simulink model "EMPlanner_cs_old"  (R2020a)
settings: Solver=ode5  StartTime=0.0  StopTime=120  FixedStep=1/1000  RelTol=1e-3
PreLoadFcn:
  | mbxruntime.callbacks.PreLoadFcn(bdroot);
PostLoadFcn:
  | mbxruntime.callbacks.PostLoadFcn(bdroot);
InitFcn:
  | mbxruntime.callbacks.InitFcn(bdroot);
StartFcn:
  | mbxruntime.callbacks.StartFcn(bdroot);
StopFcn:
  | mbxruntime.callbacks.StopFcn(bdroot);
model workspace (MAT data in the model file):
  mbox_table : object (value not decoded)
  model_closed = 0
  sim_status = 0
values from neighbouring files (symbols this model uses):
  c_factor = 43.75    [emplanner_init.m]
  cf = -175016    [emplanner_init.m]
  cr = -130634    [emplanner_init.m]
  KD_PID_distance = 0.0    (= 0)    [emplanner_init.m]
  KD_PID_speed = 0    [emplanner_init.m]
  KI_PID_distance = 0.0    (= 0)    [emplanner_init.m]
  KI_PID_speed = 0    [emplanner_init.m]
  KP_PID_distance = 0.5    [emplanner_init.m]
  KP_PID_speed = 1.8    [emplanner_init.m]
  la = 1.265    [emplanner_init.m]
  lb = 2.947-1.265    (= 1.682)    [emplanner_init.m]
  LQR_K1 = k(:,1)'    [emplanner_init.m]
  LQR_K2 = k(:,2)'    [emplanner_init.m]
  LQR_K3 = k(:,3)'    [emplanner_init.m]
  LQR_K4 = k(:,4)'    [emplanner_init.m]
  m = 2020    [emplanner_init.m]
  rack_displacement = [-39.14 , -37.2 , -35.29 , -33.43 , -31.6 , -29.81 , -28.06 , -26.34 , -24.66 ,      -23.01 , -21.38 , -19.79 , -18.23 , -16.69 , -15.18 , -13.7 , -12.23 , -10.8 , -9.38 , -7.98 ,     -6.61 , -5.25 , -3.91 , -2.59 , -1.29 , 0 , 1.27 , 2.54 , 3.78 , 5.02 , 6.24 , 7.46 , 8.66 ,      9.86 , 11.05 , 12.24 , 13.41 , 14.59 , 15.76 , 16.92 , 18.09 , 19.25 , 20.42 , 21.59 , 22.76 ,      23.93 , 25.11 , 26 ...(+26 chars)    [emplanner_init.m]
  right_wheel_ground = [-70 ,-67.2 , -64.4 , -61.6 , -58.8 , -56 , -53.2 , -50.4 , -47.6 , -44.8 , -42 ,      -39.2 , -36.4 , -33.6 , -30.8 , -28 , -25.2 , -22.4 , -19.6 , -16.8 , -14 , -11.2 , -8.4 , -5.6 ,      -2.8 , 0 , 2.8 , 5.6 , 8.4 , 11.2 , 14 , 16.8 , 19.6 , 22.4 , 25.2 , 28 , 30.8 , 33.6 , 36.4 ,      39.2 , 42 , 44.8 , 47.6 , 50.4 , 53.2 , 56 , 58.8 , 61.6 , 64.4 , 67.2 , 70 ]    [emplanner_init.m]
  vx_break_point = zeros(1,5000)    [emplanner_init.m]
undefined symbols (not defined in the file or in its folder): aubr, DiscIntNeverNeededParam, global_path_x, global_path_y, tablebr, vubr, warningInitialVelocity, x0
libraries: PreScanSimulinkLibrary x21, simulink x19, simulink_extras x6, Solver_SF x1
(part 4 of 9)

== system EMPlanner_cs_old/Audi_A8_Sedan_1/AIR_1_Demux/Activate_Switch ==
  BeamID : Inport
  Heading : Inport  Port=2
  Constant : Constant  Value=0
  Product1 : Product  RndMeth=Zero
  Relational Operator : RelationalOperator  Operator=~=  OutDataTypeStr=boolean  RndMeth=Nearest
  On/Off : Outport
  wires:
  Constant/1 -> Relational Operator/1
  Relational Operator/1 -> Product1/1
  BeamID/1 -> Relational Operator/2
  Product1/1 -> On/Off/1
  Heading/1 -> Product1/2

== system EMPlanner_cs_old/Audi_A8_Sedan_1/AIR_1_Demux/Signal2ArrayOfSignals1 ==
  note: Set mask parameter VECTORLENGTH
      |  to MAXMESSAGES
  note: Initial state of Previous vector block
      | set to zeros(VECTORLENGTH,1)
  LoopIndex : Inport
  Element : Inport  Port=2
  Assignment : Assignment  IndexOptions=Index vector (port)  Indices=1  OutputSizes=1
  Previous vector : Memory  InitialCondition=zeros(VECTORLENGTH,1)  InheritSampleTime=on
  ArrayofElements : Outport
  wires:
  Element/1 -> Assignment/2
  LoopIndex/1 -> Assignment/3
  Previous vector/1 -> Assignment/1
  Assignment/1 -> ArrayofElements/1, Previous vector/1

== system EMPlanner_cs_old/Audi_A8_Sedan_1/AIR_1_Demux/Signal2ArrayOfSignals2 ==
  note: Set mask parameter VECTORLENGTH
      |  to MAXMESSAGES
  note: Initial state of Previous vector block
      | set to zeros(VECTORLENGTH,1)
  LoopIndex : Inport
  Element : Inport  Port=2
  Assignment : Assignment  IndexOptions=Index vector (port)  Indices=1  OutputSizes=1
  Previous vector : Memory  InitialCondition=zeros(VECTORLENGTH,1)  InheritSampleTime=on
  ArrayofElements : Outport
  wires:
  Element/1 -> Assignment/2
  LoopIndex/1 -> Assignment/3
  Previous vector/1 -> Assignment/1
  Assignment/1 -> ArrayofElements/1, Previous vector/1

== system EMPlanner_cs_old/Audi_A8_Sedan_1/AIR_1_Demux/Signal2ArrayOfSignals3 ==
  note: Set mask parameter VECTORLENGTH
      |  to MAXMESSAGES
  note: Initial state of Previous vector block
      | set to zeros(VECTORLENGTH,1)
  LoopIndex : Inport
  Element : Inport  Port=2
  Assignment : Assignment  IndexOptions=Index vector (port)  Indices=1  OutputSizes=1
  Previous vector : Memory  InitialCondition=zeros(VECTORLENGTH,1)  InheritSampleTime=on
  ArrayofElements : Outport
  wires:
  Element/1 -> Assignment/2
  LoopIndex/1 -> Assignment/3
  Previous vector/1 -> Assignment/1
  Assignment/1 -> ArrayofElements/1, Previous vector/1

== system EMPlanner_cs_old/Audi_A8_Sedan_1/AIR_1_Demux/Signal2ArrayOfSignals4 ==
  note: Set mask parameter VECTORLENGTH
      |  to MAXMESSAGES
  note: Initial state of Previous vector block
      | set to zeros(VECTORLENGTH,1)
  LoopIndex : Inport
  Element : Inport  Port=2
  Assignment : Assignment  IndexOptions=Index vector (port)  Indices=1  OutputSizes=1
  Previous vector : Memory  InitialCondition=zeros(VECTORLENGTH,1)  InheritSampleTime=on
  ArrayofElements : Outport
  wires:
  Element/1 -> Assignment/2
  LoopIndex/1 -> Assignment/3
  Previous vector/1 -> Assignment/1
  Assignment/1 -> ArrayofElements/1, Previous vector/1

== system EMPlanner_cs_old/Audi_A8_Sedan_1/AIR_1_Demux/Signal2ArrayOfSignals5 ==
  note: Set mask parameter VECTORLENGTH
      |  to MAXMESSAGES
  note: Initial state of Previous vector block
      | set to zeros(VECTORLENGTH,1)
  LoopIndex : Inport
  Element : Inport  Port=2
  Assignment : Assignment  IndexOptions=Index vector (port)  Indices=1  OutputSizes=1
  Previous vector : Memory  InitialCondition=zeros(VECTORLENGTH,1)  InheritSampleTime=on
  ArrayofElements : Outport
  wires:
  Element/1 -> Assignment/2
  LoopIndex/1 -> Assignment/3
  Previous vector/1 -> Assignment/1
  Assignment/1 -> ArrayofElements/1, Previous vector/1

== system EMPlanner_cs_old/Audi_A8_Sedan_1/AIR_1_Demux/Signal2ArrayOfSignals6 ==
  note: Set mask parameter VECTORLENGTH
      |  to MAXMESSAGES
  note: Initial state of Previous vector block
      | set to zeros(VECTORLENGTH,1)
  LoopIndex : Inport
  Element : Inport  Port=2
  Assignment : Assignment  IndexOptions=Index vector (port)  Indices=1  OutputSizes=1
  Previous vector : Memory  InitialCondition=zeros(VECTORLENGTH,1)  InheritSampleTime=on
  ArrayofElements : Outport
  wires:
  Element/1 -> Assignment/2
  LoopIndex/1 -> Assignment/3
  Previous vector/1 -> Assignment/1
  Assignment/1 -> ArrayofElements/1, Previous vector/1

== system EMPlanner_cs_old/Audi_A8_Sedan_1/Dynamics_UserSpecified/CarSim2PreScanSTATE ==
  CarSim_In : Inport
  D2R : Gain  Gain=pi/180
  Demux : Demux  Outputs=[3 3 3 -1]
  Demux1 : Demux  Outputs=3
  Demux2 : Demux  Outputs=3
  Demux3 : Demux  Outputs=3
  Demux4 : Demux  Outputs=28
  Gain : Gain  Gain=9.8
  Gain1 : Gain  Gain=9.8
  Terminator_{1..26} (26 alike) : Terminator
  Transformation_SprungMassCarSim2PreScan : Subsystem
  km|h_to_m|s : Gain  Gain=1/3.6
  x [m] : Outport
  y [m] : Outport  Port=2
  z [m] : Outport  Port=3
  dx [m/s] : Outport  Port=4
  dy [m/s] : Outport  Port=5
  dz [m/s] : Outport  Port=6
  R [rad] : Outport  Port=7
  P [rad] : Outport  Port=8
  Y [rad] : Outport  Port=9
  ax[m/s^2] : Outport  Port=10
  ay[m/s^2] : Outport  Port=11
  wires:
  Demux/4 -> Demux4/1
  Demux3/3 -> Y [rad]/1
  Demux3/2 -> P [rad]/1
  Demux3/1 -> R [rad]/1
  Demux2/3 -> dz [m/s]/1
  Demux2/2 -> dy [m/s]/1
  Demux2/1 -> dx [m/s]/1
  Demux1/3 -> z [m]/1
  Demux1/2 -> y [m]/1
  Demux1/1 -> x [m]/1
  Transformation_SprungMassCarSim2PreScan/1(Out1) -> Demux1/1
  Demux/1 -> Transformation_SprungMassCarSim2PreScan/1(In1)
  CarSim_In/1 -> Demux/1
  km|h_to_m|s/1 -> Demux2/1
  Demux/2 -> km|h_to_m|s/1
  Demux/3 -> D2R/1
  D2R/1 -> Demux3/1
  Demux4/28 -> Gain1/1
  Demux4/27 -> Gain/1
  Gain/1 -> ax[m/s^2]/1
  Gain1/1 -> ay[m/s^2]/1
  Demux4/1 -> Terminator_1/1
  Demux4/2 -> Terminator_2/1
  Demux4/3 -> Terminator_3/1
  Demux4/4 -> Terminator_4/1
  Demux4/5 -> Terminator_5/1
  Demux4/6 -> Terminator_6/1
  Demux4/7 -> Terminator_7/1
  Demux4/8 -> Terminator_8/1
  Demux4/9 -> Terminator_9/1
  Demux4/10 -> Terminator_10/1
  Demux4/11 -> Terminator_11/1
  Demux4/12 -> Terminator_12/1
  Demux4/13 -> Terminator_13/1
  Demux4/14 -> Terminator_14/1
  Demux4/15 -> Terminator_15/1
  Demux4/16 -> Terminator_16/1
  Demux4/17 -> Terminator_17/1
  Demux4/18 -> Terminator_18/1
  Demux4/19 -> Terminator_19/1
  Demux4/20 -> Terminator_20/1
  Demux4/21 -> Terminator_21/1
  Demux4/22 -> Terminator_22/1
  Demux4/23 -> Terminator_23/1
  Demux4/24 -> Terminator_24/1
  Demux4/25 -> Terminator_25/1
  Demux4/26 -> Terminator_26/1

== system EMPlanner_cs_old/Audi_A8_Sedan_1/Dynamics_UserSpecified/MuxState ==
  note: mode: Dynamics
  note: mode: Positioning
  note: mode: Dynamics
      | VelVEHICLE
      | wrt VEH
  note: AnglesVEHICLE
      | wrtGLOB
  note: For state mode 'Dynamic' positions
      | are not taken into account, as they
      | are computed by integrating velocity.
      | Click annotation for Help.
  x [m] : Inport  SampleTime=TimeStep
  y [m] : Inport  Port=2  SampleTime=TimeStep
  z [m] : Inport  Port=3  SampleTime=TimeStep
  dx [m/s] : Inport  Port=4  SampleTime=TimeStep
  dy [m/s] : Inport  Port=5  SampleTime=TimeStep
  dz [m/s] : Inport  Port=6  SampleTime=TimeStep
  R [rad] : Inport  Port=7  SampleTime=TimeStep
  P [rad] : Inport  Port=8  SampleTime=TimeStep
  Y [rad] : Inport  Port=9  SampleTime=TimeStep
  Constant : Constant  DisableCoverage=on  Value=positioningmode
  Discrete-Time Integrator : DiscreteIntegrator  SampleTime=TimeStep  ICPrevOutput=DiscIntNeverNeededParam  ICPrevScaledInput=DiscIntNeverNeededParam
  Ground : Ground
  Ground1 : Ground
  Mux1 : Mux  Inputs=[3 3]
  Mux2 : Mux  Inputs=3
  Mux3 : Mux  Inputs=3
  Mux4 : Mux  Inputs=3
  Mux5 : Mux  Inputs=[3 3]
  Mux6 : Mux  Inputs=[6 3]
  Switch : Switch  Threshold=0.5
  Transformation_BODY2GLOBAL : PreScanSimulinkLibrary/Simple_Vehicle_Dynamics/Chassis/MuxDynState/Transformation_BODY2GLOBAL  SystemSampleTime=-1  Latency=0  AutoFrameSizeCalculation=off
  mux3 : Mux  Inputs=3
  state : Outport
  wires:
  Constant/1 -> Switch/2
  Mux6/1 -> state/1
  Mux4/1 -> Mux1/1
  Mux5/1 -> Switch/3
  Mux1/1 -> Switch/1
  Switch/1 -> Mux6/1  "PosVeh wrt  GLOB"
  P [rad]/1 -> Mux3/2
  R [rad]/1 -> Mux3/1
  dz [m/s]/1 -> Mux2/3
  dy [m/s]/1 -> Mux2/2
  dx [m/s]/1 -> Mux2/1
  z [m]/1 -> Mux4/3
  y [m]/1 -> Mux4/2
  x [m]/1 -> Mux4/1
  Ground1/1 -> mux3/2  "pitch"
  Y [rad]/1 -> mux3/3, Mux3/3  "yaw"
  Mux3/1 -> Mux6/2
  Transformation_BODY2GLOBAL/1 -> Discrete-Time Integrator/1, Mux5/2  "VelVEH wrt  GLOB"
  mux3/1 -> Transformation_BODY2GLOBAL/2
  Ground/1 -> mux3/1  "roll"
  Mux2/1 -> Mux1/2, Transformation_BODY2GLOBAL/1
  Discrete-Time Integrator/1 -> Mux5/1  "PosVEH wrt  GLOB"

== system EMPlanner_cs_old/Audi_A8_Sedan_1/SELF_Demux/compas converter ==
  rotz [rad] : Inport
  cart2compas : Subsystem
  rad2deg : Gain  Gain=180/pi
  heading [deg] : Outport
  wires:
  rad2deg/1 -> cart2compas/1(Angle [deg])
  rotz [rad]/1 -> rad2deg/1
  cart2compas/1(heading [deg]) -> heading [deg]/1

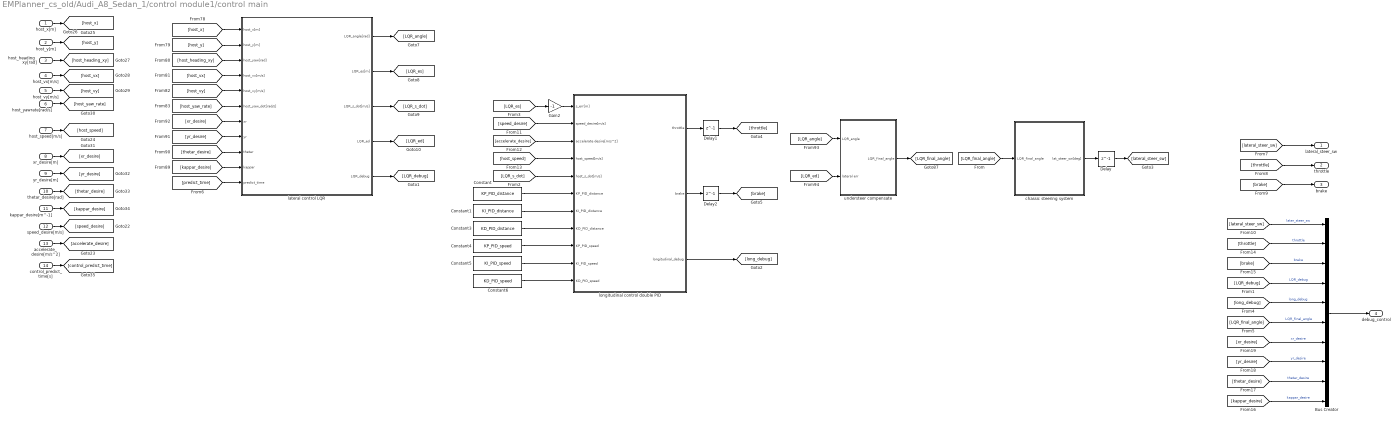
== system EMPlanner_cs_old/Audi_A8_Sedan_1/control module1/control main ==
  host_x[m] : Inport
  host_y[m] : Inport  Port=2
  host_heading_xy[rad] : Inport  Port=3
  host_vx[m/s] : Inport  Port=4
  host_vy[m/s] : Inport  Port=5
  host_yawrate[rad/s] : Inport  Port=6
  host_speed[m/s] : Inport  Port=7
  xr_desire[m] : Inport  Port=8
  yr_desire[m] : Inport  Port=9
  thetar_desire[rad] : Inport  Port=10
  kappar_desire[m^-1] : Inport  Port=11
  speed_desire[m/s] : Inport  Port=12
  accelerate_desire[m/s^2] : Inport  Port=13
  control_predict_time[s] : Inport  Port=14
  Bus Creator : BusCreator  Inputs=10
  Constant : Constant  Value=KP_PID_distance
  Constant1 : Constant  Value=KI_PID_distance
  Constant3 : Constant  Value=KD_PID_distance
  Constant4 : Constant  Value=KP_PID_speed
  Constant5 : Constant  Value=KI_PID_speed
  Constant6 : Constant  Value=KD_PID_speed
  Delay : Delay  DelayLength=1
  Delay1 : Delay  DelayLength=1
  Delay2 : Delay  DelayLength=1
  Gain2 : Gain  Gain=-1
  chassic steering system : Subsystem
  lateral control LQR : Subsystem
  longitudinal control double PID : Subsystem
  understeer compensate : Subsystem
  lateral_steer_sw : Outport
  throttle : Outport  Port=2
  brake : Outport  Port=3
  debug_control : Outport  Port=4
  wires:
  host_x[m]/1 -> [host_x]
  understeer compensate/1(LQR_final_angle) -> [LQR_final_angle]
  lateral control LQR/1(LQR_angle[rad]) -> [LQR_angle]
  [host_vx] -> lateral control LQR/4(host_vx[m/s])
  thetar_desire[rad]/1 -> [thetar_desire]
  Constant1/1 -> longitudinal control double PID/7(KI_PID_distance)
  [accelerate_desire] -> longitudinal control double PID/3(accelerate desire[m/s^2])
  [host_x] -> lateral control LQR/1(host_x[m])
  [xr_desire] -> lateral control LQR/7(xr)
  accelerate_desire[m/s^2]/1 -> [accelerate_desire]
  [host_y] -> lateral control LQR/2(host_y[m])
  [LQR_s_dot] -> longitudinal control double PID/5(host_s_dot[m/s])
  [yr_desire] -> lateral control LQR/8(yr)
  [LQR_angle] -> understeer compensate/1(LQR_angle)
  xr_desire[m]/1 -> [xr_desire]
  [host_vy] -> lateral control LQR/5(host_vy[m/s])
  lateral control LQR/2(LQR_es[m]) -> [LQR_es]
  host_heading_xy[rad]/1 -> [host_heading_xy]
  [LQR_ed] -> understeer compensate/2(lateral err)
  lateral control LQR/3(LQR_s_dot[m/s]) -> [LQR_s_dot]
  Constant/1 -> longitudinal control double PID/6(KP_PID_distance)
  Constant3/1 -> longitudinal control double PID/8(KD_PID_distance)
  Constant5/1 -> longitudinal control double PID/10(KI_PID_speed)
  Constant4/1 -> longitudinal control double PID/9(KP_PID_speed)
  [host_speed] -> longitudinal control double PID/4(host_speed[m/s])
  [predict_time] -> lateral control LQR/11(predict_time)
  host_vx[m/s]/1 -> [host_vx]
  [speed_desire] -> longitudinal control double PID/2(speed_desire[m/s])
  lateral control LQR/4(LQR_ed) -> [LQR_ed]
  [thetar_desire] -> lateral control LQR/9(thetar)
  [host_heading_xy] -> lateral control LQR/3(host_yaw[rad])
  [kappar_desire] -> lateral control LQR/10(kappar)
  host_yawrate[rad/s]/1 -> [host_yaw_rate]
  kappar_desire[m^-1]/1 -> [kappar_desire]
  yr_desire[m]/1 -> [yr_desire]
  [host_yaw_rate] -> lateral control LQR/6(host_yaw_dot[rad/s])
  host_y[m]/1 -> [host_y]
  host_vy[m/s]/1 -> [host_vy]
  host_speed[m/s]/1 -> [host_speed]
  control_predict_time[s]/1 -> [control_predict_time]
  speed_desire[m/s]/1 -> [speed_desire]
  Constant6/1 -> longitudinal control double PID/11(KD_PID_speed)
  Gain2/1 -> longitudinal control double PID/1(s_err[m])
  [LQR_es] -> Gain2/1
  [LQR_final_angle] -> chassic steering system/1(LQR_final_angle)
  chassic steering system/1(lat_steer_sw[deg]) -> Delay/1
  longitudinal control double PID/1(throttle) -> Delay1/1
  longitudinal control double PID/2(brake) -> Delay2/1
  lateral control LQR/5(LQR_debug) -> [LQR_debug]
  longitudinal control double PID/3(longitudinal_debug) -> [long_debug]
  Delay/1 -> [lateral_steer_sw]
  Delay1/1 -> [throttle]
  Delay2/1 -> [brake]
  [lateral_steer_sw] -> lateral_steer_sw/1
  [throttle] -> throttle/1
  [brake] -> brake/1
  [lateral_steer_sw] -> Bus Creator/1  "later_steer_sw"
  [throttle] -> Bus Creator/2  "throttle"
  [brake] -> Bus Creator/3  "brake"
  [LQR_debug] -> Bus Creator/4  "LQR_debug"
  [long_debug] -> Bus Creator/5  "long_debug"
  [LQR_final_angle] -> Bus Creator/6  "LQR_final_angle"
  Bus Creator/1 -> debug_control/1
  [xr_desire] -> Bus Creator/7  "xr_desire"
  [yr_desire] -> Bus Creator/8  "yr_desire"
  [thetar_desire] -> Bus Creator/9  "thetar_desire"
  [kappar_desire] -> Bus Creator/10  "kappar_desire"

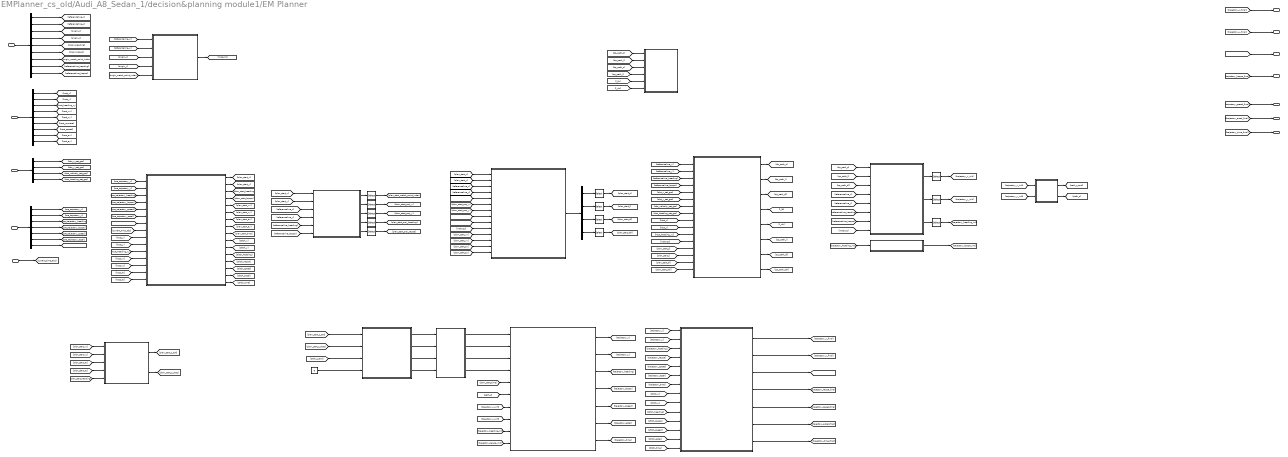
== system EMPlanner_cs_old/Audi_A8_Sedan_1/decision&planning module1/EM Planner ==
  referenceline info : Inport
  location info : Inport  Port=2
  perception info : Inport  Port=3
  pre_planning info : Inport  Port=4
  current_time_abs : Inport  Port=5
  Bus Selector : BusSelector  OutputSignals=trajectory_x,trajectory_y,trajectory_heading,trajectory_kappa,trajectory_speed,trajectory_accel,trajectory_time_abs
  Bus Selector1 : BusSelector  OutputSignals=referenceline_x,referenceline_y,origin_x,origin_y,origin_heading,origin_kappa,origin_match_point_index,referenceline_heading,referenceline_kappa
  Bus Selector2 : BusSelector  OutputSignals=obs_x_set_gcs,obs_y_set_gcs,obs_velocity_set_gcs,obs_heading_set_gcs
  Bus Selector3 : BusSelector  OutputSignals=host_x,host_y,host_heading_xy,host_vx,host_vy,host_yawrate,host_speed,host_ax,host_ay
  Bus Selector4 : BusSelector  OutputSignals=s_set,l_set,dl_set,ddl_set
  Constant1 : Constant  Value=8
  General Cartesian2Frenet : Subsystem
  MATLAB Function : MATLAB Function  TreatAsAtomicUnit=on
  MATLAB Function1 : MATLAB Function  TreatAsAtomicUnit=on
  MATLAB Function2 : MATLAB Function  TreatAsAtomicUnit=on
  MATLAB Function3 : MATLAB Function  TreatAsAtomicUnit=on
  MATLAB Function4 : MATLAB Function  TreatAsAtomicUnit=on
  MATLAB Function5 : MATLAB Function  TreatAsAtomicUnit=on
  MATLAB Function6 : MATLAB Function  TreatAsAtomicUnit=on
  MATLAB Function7 : MATLAB Function  TreatAsAtomicUnit=on
  MATLAB Function8 : MATLAB Function  TreatAsAtomicUnit=on
  MATLAB Function9 : MATLAB Function  TreatAsAtomicUnit=on
  Selector : Selector  InputPortWidth=128  IndexOptions=Index vector (dialog)  Indices=[1:120]  OutputSizes=1
  Selector1 : Selector  InputPortWidth=128  IndexOptions=Index vector (dialog)  Indices=[1:120]  OutputSizes=1
  Selector{6..10} (5 alike) : Selector  InputPortWidth=128  IndexOptions=Index vector (dialog)  Indices=1  OutputSizes=1
  Selector{11..14} (4 alike) : Selector  InputPortWidth=128  IndexOptions=Index vector (dialog)  Indices=[1]  OutputSizes=1
  Selector2 : Selector  InputPortWidth=128  IndexOptions=Index vector (dialog)  Indices=[1:120]  OutputSizes=1
  calc plan start gcs : MATLAB Function  TreatAsAtomicUnit=on
  generate index to s : MATLAB Function  TreatAsAtomicUnit=on
  path decision and planning : Subsystem
  trajectory_x : Outport
  trajectory_y : Outport  Port=2
  trajectory_heading : Outport  Port=3
  trajectory_kappa : Outport  Port=4
  trajectory_speed : Outport  Port=5
  trajectory_accel : Outport  Port=6
  trajectoty_time : Outport  Port=7
  wires:
  Bus Selector3/2 -> [host_y]  "<host_y>"
  Bus Selector1/1 -> [referenceline_x]  "<referenceline_x>"
  Bus Selector1/5 -> [origin_heading]  "<origin_heading>"
  Bus Selector1/3 -> [origin_x]  "<origin_x>"
  Bus Selector1/2 -> [referenceline_y]  "<referenceline_y>"
  Bus Selector3/4 -> [host_vx]  "<host_vx>"
  [origin_x] -> generate index to s/3(origin_x)
  [referenceline_y] -> generate index to s/2(path_y)
  Bus Selector3/9 -> [host_ay]  "<host_ay>"
  location info/1 -> Bus Selector3/1
  Bus Selector3/1 -> [host_x]  "<host_x>"
  [origin_match_point_index] -> generate index to s/5(origin_match_point_index)
  Bus Selector3/8 -> [host_ax]  "<host_ax>"
  [origin_y] -> generate index to s/4(origin_y)
  Bus Selector3/3 -> [host_heading_xy]  "<host_heading_xy>"
  Bus Selector3/7 -> [host_speed]  "<host_speed>"
  Bus Selector3/6 -> [host_yawrate]  "<host_yawrate>"
  Bus Selector3/5 -> [host_vy]  "<host_vy>"
  Bus Selector1/7 -> [origin_match_point_index]  "<origin_match_point_index>"
  Bus Selector1/6 -> [origin_kappa]  "<origin_kappa>"
  Bus Selector1/4 -> [origin_y]  "<origin_y>"
  [referenceline_x] -> generate index to s/1(path_x)
  generate index to s/1(index2s) -> [index2s]
  referenceline info/1 -> Bus Selector1/1
  Bus Selector2/3 -> [obs_velocity_set_gcs]  "<obs_velocity_set_gcs>"
  perception info/1 -> Bus Selector2/1
  Bus Selector2/4 -> [obs_heading_set_gcs]  "<obs_heading_set_gcs>"
  Bus Selector2/1 -> [obs_x_set_gcs]  "<obs_x_set_gcs>"
  Bus Selector2/2 -> [obs_y_set_gcs]  "<obs_y_set_gcs>"
  pre_planning info/1 -> Bus Selector/1
  Bus Selector1/8 -> [referenceline_heading]  "<referenceline_heading>"
  Bus Selector1/9 -> [referenceline_kappa]  "<referenceline_kappa>"
  [index2s] -> path decision and planning/12(index2s)
  [referenceline_x] -> path decision and planning/1(referenceline_x)
  [referenceline_y] -> path decision and planning/2(referenceline_y)
  [referenceline_heading] -> path decision and planning/3(referenceline_heading)
  [referenceline_kappa] -> path decision and planning/4(referenceline_kappa)
  [obs_x_set_gcs] -> path decision and planning/5(obs_x_set_gcs)
  [obs_y_set_gcs] -> path decision and planning/6(obs_y_set_gcs)
  [obs_velocity_set_gcs] -> path decision and planning/7(obs_velocity_set_gcs)
  [obs_heading_set_gcs] -> path decision and planning/8(obs_heading_set_gcs)
  [host_heading_xy] -> path decision and planning/11(host_heading_xy)
  [host_y] -> path decision and planning/10(host_y)
  [host_x] -> path decision and planning/9(host_x)
  path decision and planning/1(dp_path_s) -> [dp_path_s]
  path decision and planning/2(dp_path_l) -> [dp_path_l]
  path decision and planning/3(dp_path_dl) -> [dp_path_dl]
  [dp_path_l] -> MATLAB Function1/2(qp_path_l)
  [dp_path_s] -> MATLAB Function1/1(qp_path_s)
  path decision and planning/4(l_lb) -> [l_lb]
  path decision and planning/5(l_ub) -> [l_ub]
  [l_ub] -> MATLAB Function1/6(l_ub)
  [l_lb] -> MATLAB Function1/5(l_lb)
  path decision and planning/6(qp_path_l) -> [qp_path_l]
  [qp_path_l] -> MATLAB Function1/4(dp_path_l)
  [dp_path_s] -> MATLAB Function1/3(dp_path_s)
  path decision and planning/7(qp_path_dl) -> [qp_path_dl]
  current_time_abs/1 -> [current_time_abs]
  Selector/1 -> [trajectory_x_init]
  Selector1/1 -> [trajectory_y_init]
  Selector2/1 -> [trajectory_heading_init]
  [qp_path_dl] -> MATLAB Function3/3(dl_set)
  [dp_path_s] -> MATLAB Function3/1(s_set)
  [qp_path_l] -> MATLAB Function3/2(l_set)
  [referenceline_x] -> MATLAB Function3/4(frenet_path_x)
  [referenceline_y] -> MATLAB Function3/5(frenet_path_y)
  [referenceline_heading] -> MATLAB Function3/6(frenet_path_heading)
  [referenceline_kappa] -> MATLAB Function3/7(frenet_path_kappa)
  [index2s] -> MATLAB Function3/8(index2s)
  MATLAB Function3/1(x_set) -> Selector/1
  MATLAB Function3/2(y_set) -> Selector1/1
  MATLAB Function3/3(theta_set) -> Selector2/1
  [trajectory_heading_init] -> MATLAB Function/1(trajectory_heading)
  MATLAB Function/1(trajectory_kappa) -> [trajectory_kappa_init]
  Bus Selector/1 -> [pre_trajectory_x]  "<trajectory_x>"
  Bus Selector/2 -> [pre_trajectory_y]  "<trajectory_y>"
  Bus Selector/3 -> [pre_trajectory_heading]  "<trajectory_heading>"
  Bus Selector/4 -> [pre_trajectory_kappa]  "<trajectory_kappa>"
  Bus Selector/5 -> [pre_trajectory_speed]  "<trajectory_speed>"
  Bus Selector/6 -> [pre_trajectory_accel]  "<trajectory_accel>"
  Bus Selector/7 -> [pre_trajectory_time_abs]  "<trajectory_time_abs>"
  [current_time_abs] -> calc plan start gcs/8(current_time)
  [host_y] -> calc plan start gcs/10(host_y)
  [host_x] -> calc plan start gcs/9(host_x)
  [pre_trajectory_x] -> calc plan start gcs/1(pre_trajectory_x)
  [pre_trajectory_y] -> calc plan start gcs/2(pre_trajectory_y)
  [pre_trajectory_heading] -> calc plan start gcs/3(pre_trajectory_heading)
  [pre_trajectory_kappa] -> calc plan start gcs/4(pre_trajectory_kappa)
  [pre_trajectory_speed] -> calc plan start gcs/5(pre_trajectory_velocity)
  [pre_trajectory_accel] -> calc plan start gcs/6(pre_trajectory_accel)
  [pre_trajectory_time_abs] -> calc plan start gcs/7(pre_trajectory_time_abs)
  [host_heading_xy] -> calc plan start gcs/11(host_heading_xy)
  [host_vx] -> calc plan start gcs/12(host_vx)
  [host_vy] -> calc plan start gcs/13(host_vy)
  [host_ax] -> calc plan start gcs/14(host_ax)
  [host_ay] -> calc plan start gcs/15(host_ay)
  calc plan start gcs/1(plan_start_x) -> [plan_start_x]
  calc plan start gcs/2(plan_start_y) -> [plan_start_y]
  calc plan start gcs/3(plan_start_heading) -> [plan_start_heading]
  calc plan start gcs/4(plan_start_kappa) -> [plan_start_kappa]
  calc plan start gcs/5(plan_start_vx) -> [plan_start_vx]
  calc plan start gcs/6(plan_start_vy) -> [plan_start_vy]
  calc plan start gcs/7(plan_start_ax) -> [plan_start_ax]
  calc plan start gcs/8(plan_start_ay) -> [plan_start_ay]
  calc plan start gcs/10(stitch_x) -> [stitch_x]
  calc plan start gcs/11(stitch_y) -> [stitch_y]
  calc plan start gcs/12(stitch_heading) -> [stitch_heading]
  calc plan start gcs/13(stitch_kappa) -> [stitch_kappa]
  calc plan start gcs/14(stitch_speed) -> [stitch_speed]
  calc plan start gcs/15(stitch_accel) -> [stitch_accel]
  calc plan start gcs/16(stitch_time) -> [stitch_time]
  [referenceline_kappa] -> MATLAB Function2/6(frenet_path_kappa)
  [referenceline_heading] -> MATLAB Function2/5(frenet_path_heading)
  [referenceline_y] -> MATLAB Function2/4(frenet_path_y)
  [referenceline_x] -> MATLAB Function2/3(frenet_path_x)
  [plan_start_y] -> MATLAB Function2/2(y_set)
  [plan_start_x] -> MATLAB Function2/1(x_set)
  MATLAB Function2/1(match_point_index_set) -> Selector6/1
  MATLAB Function2/2(proj_x_set) -> Selector7/1
  MATLAB Function2/3(proj_y_set) -> Selector8/1
  MATLAB Function2/4(proj_heading_set) -> Selector9/1
  MATLAB Function2/5(proj_kappa_set) -> Selector10/1
  Selector6/1 -> [plan_start_match_point_index]
  Selector7/1 -> [plan_start_proj_x]
  Selector8/1 -> [plan_start_proj_y]
  Selector9/1 -> [plan_start_proj_heading]
  Selector10/1 -> [plan_start_proj_kappa]
  [plan_start_match_point_index] -> General Cartesian2Frenet/5(proj_match_point_index_set)
  [plan_start_proj_x] -> General Cartesian2Frenet/6(proj_x_set)
  [plan_start_proj_y] -> General Cartesian2Frenet/7(proj_y_set)
  [plan_start_proj_heading] -> General Cartesian2Frenet/8(proj_heading_set)
  [plan_start_proj_kappa] -> General Cartesian2Frenet/9(proj_kappa_set)
  [index2s] -> General Cartesian2Frenet/10(index2s)
  [plan_start_vx] -> General Cartesian2Frenet/11(vx_set)
  [plan_start_vy] -> General Cartesian2Frenet/12(vy_set)
  [plan_start_ax] -> General Cartesian2Frenet/13(ax_set)
  [plan_start_ay] -> General Cartesian2Frenet/14(ay_set)
  [referenceline_y] -> General Cartesian2Frenet/4(frenet_path_y)
  [referenceline_x] -> General Cartesian2Frenet/3(frenet_path_x)
  [plan_start_y] -> General Cartesian2Frenet/2(y_set)
  [plan_start_x] -> General Cartesian2Frenet/1(x_set)
  Selector12/1 -> [plan_start_l]
  Selector14/1 -> [plan_start_ddl]
  Bus Selector4/2 -> Selector12/1  "<l_set>"
  Selector13/1 -> [plan_start_dl]
  Selector11/1 -> [plan_start_s]
  Bus Selector4/3 -> Selector13/1  "<dl_set>"
  Bus Selector4/4 -> Selector14/1  "<ddl_set>"
  Bus Selector4/1 -> Selector11/1  "<s_set>"
  General Cartesian2Frenet/1(Carte2FrenetOut) -> Bus Selector4/1
  [plan_start_s] -> path decision and planning/13(plan_start_s)
  [plan_start_l] -> path decision and planning/14(plan_start_l)
  [plan_start_dl] -> path decision and planning/15(plan_start_dl)
  [plan_start_ddl] -> path decision and planning/16(plan_start_ddl)
  calc plan start gcs/9(plan_start_time) -> [plan_start_time]
  [plan_start_vx] -> MATLAB Function4/1(plan_start_vx)
  [plan_start_vy] -> MATLAB Function4/2(plan_start_vy)
  [plan_start_ax] -> MATLAB Function4/3(plan_start_ax)
  [plan_start_ay] -> MATLAB Function4/4(plan_start_ay)
  [plan_start_heading] -> MATLAB Function4/5(plan_start_heading)
  MATLAB Function4/1(plan_start_s_dot) -> [plan_start_s_dot]
  MATLAB Function4/2(plan_start_s_dot2) -> [plan_start_s_dot2]
  [plan_start_s_dot] -> MATLAB Function6/1(plan_start_s_dot)
  [plan_start_s_dot2] -> MATLAB Function6/2(plan_start_s_dot2)
  Constant1/1 -> MATLAB Function6/4(recommend_T)
  MATLAB Function5/1(path_s_end) -> [path_s_end]
  path decision and planning/8(qp_path_ddl) -> [qp_path_ddl]
  MATLAB Function5/2(path_s) -> [path_s]
  [trajectory_x_init] -> MATLAB Function5/1(trajectory_x)
  [trajectory_y_init] -> MATLAB Function5/2(trajectory_y)
  [path_s] -> MATLAB Function7/6(path_s)
  [trajectory_x_init] -> MATLAB Function7/7(trajectory_x_init)
  [trajectory_y_init] -> MATLAB Function7/8(trajectory_y_init)
  [trajectory_heading_init] -> MATLAB Function7/9(trajectory_heading_init)
  [trajectory_kappa_init] -> MATLAB Function7/10(trajectory_kappa_init)
  MATLAB Function7/1(trajectory_x) -> [trajectory_x]
  MATLAB Function7/2(trajectory_y) -> [trajectory_y]
  MATLAB Function7/3(trajectory_heading) -> [trajectory_heading]
  MATLAB Function7/4(trajectory_kappa) -> [trajectory_kappa]
  MATLAB Function7/5(trajectory_speed) -> [trajectory_speed]
  MATLAB Function7/6(trajectory_accel) -> [trajectory_accel]
  MATLAB Function7/7(trajectory_time) -> [trajectory_time]
  [path_s_end] -> MATLAB Function6/3(s_end)
  [trajectory_x] -> MATLAB Function8/1(trajectory_x)
  [trajectory_y] -> MATLAB Function8/2(trajectory_y)
  [trajectory_heading] -> MATLAB Function8/3(trajectory_heading)
  [trajectory_kappa] -> MATLAB Function8/4(trajectory_kappa)
  [trajectory_speed] -> MATLAB Function8/5(trajectory_speed)
  [trajectory_accel] -> MATLAB Function8/6(trajectory_accel)
  [trajectory_time] -> MATLAB Function8/7(trajectory_time)
  [stitch_x] -> MATLAB Function8/8(stitch_x)
  [stitch_y] -> MATLAB Function8/9(stitch_y)
  [stitch_heading] -> MATLAB Function8/10(stitch_heading)
  [stitch_kappa] -> MATLAB Function8/11(stitch_kappa)
  [stitch_speed] -> MATLAB Function8/12(stitch_speed)
  [stitch_accel] -> MATLAB Function8/13(stitch_accel)
  [stitch_time] -> MATLAB Function8/14(stitch_time)
  [plan_start_time] -> MATLAB Function7/5(current_time)
  MATLAB Function8/1(trajectory_x_final) -> [trajectory_x_final]
  MATLAB Function8/2(trajectory_y_final) -> [trajectory_y_final]
  MATLAB Function8/3(trajectory_heading_final) -> [trajectory_heading_final]
  MATLAB Function8/4(trajectory_kappa_final) -> [trajectory_kappa_final]
  MATLAB Function8/5(trajectory_speed_final) -> [trajectory_speed_final]
  MATLAB Function8/6(trajectory_accel_final) -> [trajectory_accel_final]
  MATLAB Function8/7(trajectory_time_final) -> [trajectory_time_final]
  [trajectory_x_final] -> trajectory_x/1
  [trajectory_y_final] -> trajectory_y/1
  [trajectory_heading_final] -> trajectory_heading/1
  [trajectory_time_final] -> trajectoty_time/1
  [trajectory_accel_final] -> trajectory_accel/1
  [trajectory_speed_final] -> trajectory_speed/1
  [trajectory_kappa_final] -> trajectory_kappa/1
  MATLAB Function6/1(s_init) -> MATLAB Function9/1(s_init)
  MATLAB Function6/2(s_dot_init) -> MATLAB Function9/2(s_dot_init)
  MATLAB Function6/3(s_dot2_init) -> MATLAB Function9/3(s_dot2_init)
  MATLAB Function6/4(relative_time_init) -> MATLAB Function9/4(relative_time_init)
  MATLAB Function9/1(s) -> MATLAB Function7/1(s)
  MATLAB Function9/2(s_dot) -> MATLAB Function7/2(s_dot)
  MATLAB Function9/3(s_dot2) -> MATLAB Function7/3(s_dot2)
  MATLAB Function9/4(relative_time) -> MATLAB Function7/4(relative_time)

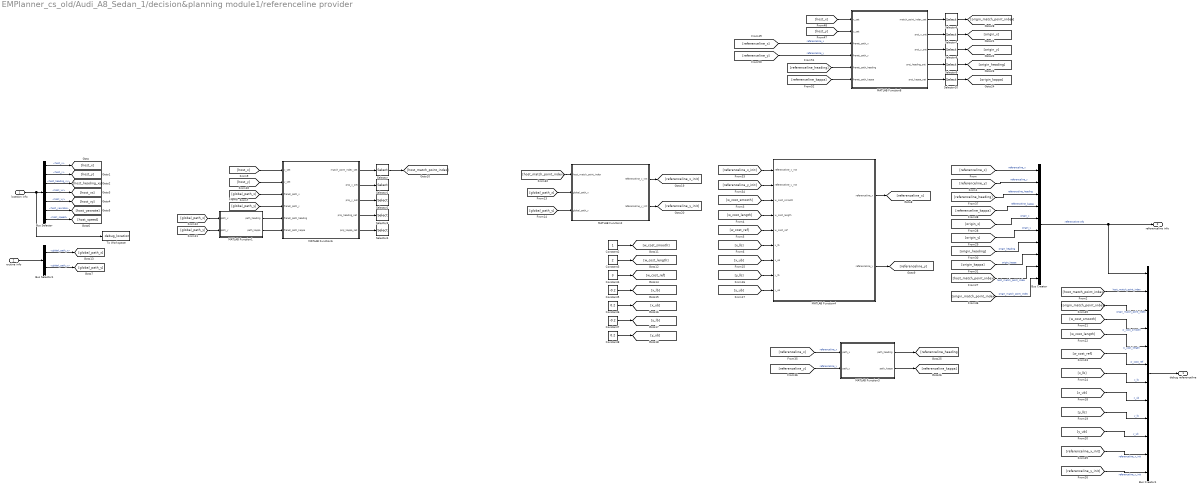
== system EMPlanner_cs_old/Audi_A8_Sedan_1/decision&planning module1/referenceline provider ==
  location info : Inport
  routine info : Inport  Port=2
  Bus Creator : BusCreator  Inputs=10
  Bus Creator1 : BusCreator  Inputs=12
  Bus Selector : BusSelector  OutputSignals=host_x,host_y,host_heading_xy,host_vx,host_vy,host_yawrate,host_speed
  Bus Selector1 : BusSelector  OutputSignals=global_path_x,global_path_y
  Constant2 : Constant
  Constant3 : Constant  Value=2
  Constant4 : Constant  Value=3
  Constant5 : Constant  Value=-0.2
  Constant6 : Constant  Value=0.2
  Constant7 : Constant  Value=-0.2
  Constant8 : Constant  Value=0.2
  MATLAB Function1 : MATLAB Function  TreatAsAtomicUnit=on
  MATLAB Function2 : MATLAB Function  TreatAsAtomicUnit=on
  MATLAB Function3 : MATLAB Function  TreatAsAtomicUnit=on
  MATLAB Function4 : MATLAB Function  TreatAsAtomicUnit=on
  MATLAB Function6 : MATLAB Function  TreatAsAtomicUnit=on
  MATLAB Function8 : MATLAB Function  TreatAsAtomicUnit=on
  Selector{,1..4,6..10} (10 alike) : Selector  InputPortWidth=128  IndexOptions=Index vector (dialog)  Indices=1  OutputSizes=1
  To Workspace : ToWorkspace  VariableName=debug_location  SaveFormat=Timeseries  SampleTime=-1
  debug referenceline : Outport
  referenceline info : Outport  Port=2
  wires:
  [global_path_x] -> MATLAB Function2/2(global_path_x)
  [host_x] -> MATLAB Function6/1(x_set)
  MATLAB Function1/2(path_kappa) -> MATLAB Function6/6(frenet_path_kappa)
  MATLAB Function1/1(path_heading) -> MATLAB Function6/5(frenet_path_heading)
  [global_path_y] -> MATLAB Function6/4(frenet_path_y)
  [global_path_x] -> MATLAB Function6/3(frenet_path_x)
  [host_y] -> MATLAB Function6/2(y_set)
  [global_path_y] -> MATLAB Function1/2(path_y)
  [global_path_x] -> MATLAB Function1/1(path_x)
  [global_path_y] -> MATLAB Function2/3(global_path_y)
  MATLAB Function2/1(referenceline_x_init) -> [referenceline_x_init]
  Bus Selector/5 -> [host_vy]  "<host_vy>"
  Bus Selector/1 -> [host_x]  "<host_x>"
  Bus Selector/2 -> [host_y]  "<host_y>"
  Bus Selector/3 -> [host_heading_xy]  "<host_heading_xy>"
  Bus Selector/4 -> [host_vx]  "<host_vx>"
  Bus Selector/7 -> [host_speed]  "<host_speed>"
  Bus Selector/6 -> [host_yawrate]  "<host_yawrate>"
  location info/1 -> To Workspace/1, Bus Selector/1
  Bus Selector1/2 -> [global_path_y]  "<global_path_y>"
  Bus Selector1/1 -> [global_path_x]  "<global_path_x>"
  routine info/1 -> Bus Selector1/1
  MATLAB Function4/1(referenceline_x) -> [referenceline_x]
  MATLAB Function4/2(referenceline_y) -> [referenceline_y]
  [referenceline_x] -> Bus Creator/1  "referenceline_x"
  [referenceline_y] -> Bus Creator/2  "referenceline_y"
  Bus Creator1/1 -> debug referenceline/1
  Bus Creator/1 -> Bus Creator1/1, referenceline info/1  "referenceline info"
  Constant2/1 -> [w_cost_smooth]
  Constant3/1 -> [w_cost_length]
  Constant8/1 -> [y_ub]
  Constant7/1 -> [y_lb]
  Constant6/1 -> [x_ub]
  Constant5/1 -> [x_lb]
  Constant4/1 -> [w_cost_ref]
  [w_cost_smooth] -> MATLAB Function4/3(w_cost_smooth)
  [w_cost_length] -> MATLAB Function4/4(w_cost_length)
  [w_cost_ref] -> MATLAB Function4/5(w_cost_ref)
  [x_lb] -> MATLAB Function4/6(x_lb)
  [x_ub] -> MATLAB Function4/7(x_ub)
  [y_lb] -> MATLAB Function4/8(y_lb)
  [y_ub] -> MATLAB Function4/9(y_ub)
  [w_cost_ref] -> Bus Creator1/6  "w_cost_ref"
  [x_lb] -> Bus Creator1/7  "x_lb"
  [w_cost_length] -> Bus Creator1/5  "w_cost_length"
  [x_ub] -> Bus Creator1/8  "x_ub"
  [w_cost_smooth] -> Bus Creator1/4  "w_cost_smooth"
  [y_lb] -> Bus Creator1/9  "y_lb"
  [host_match_point_index] -> Bus Creator1/2  "host_match_point_index"
  [y_ub] -> Bus Creator1/10  "y_ub"
  [referenceline_x_init] -> Bus Creator1/11  "referenceline_x_init"
  [referenceline_y_init] -> Bus Creator1/12  "referenceline_y_init"
  MATLAB Function6/1(match_point_index_set) -> Selector/1
  MATLAB Function6/2(proj_x_set) -> Selector1/1
  MATLAB Function6/3(proj_y_set) -> Selector2/1
  MATLAB Function6/4(proj_heading_set) -> Selector3/1
  MATLAB Function6/5(proj_kappa_set) -> Selector4/1
  [origin_x] -> Bus Creator/5  "origin_x"
  [origin_y] -> Bus Creator/6  "origin_y"
  [origin_heading] -> Bus Creator/7  "origin_heading"
  [origin_kappa] -> Bus Creator/8  "origin_kappa"
  [host_match_point_index] -> Bus Creator/9  "host_match_point_index"
  [host_match_point_index] -> MATLAB Function2/1(host_match_point_index)
  MATLAB Function2/2(referenceline_y_init) -> [referenceline_y_init]
  [referenceline_x_init] -> MATLAB Function4/1(referenceline_x_init)
  [referenceline_y_init] -> MATLAB Function4/2(referenceline_y_init)
  [referenceline_y] -> MATLAB Function3/2(path_y)  "referenceline_y"
  [referenceline_x] -> MATLAB Function3/1(path_x)  "referenceline_x"
  MATLAB Function3/1(path_heading) -> [referenceline_heading]
  MATLAB Function3/2(path_kappa) -> [referenceline_kappa]
  [referenceline_heading] -> Bus Creator/3  "referenceline_heading"
  [referenceline_kappa] -> Bus Creator/4  "referenceline_kappa"
  [origin_match_point_index] -> Bus Creator1/3  "origin_match_point_index"
  [origin_match_point_index] -> Bus Creator/10  "origin_match_point_index"
  MATLAB Function8/5(proj_kappa_set) -> Selector10/1
  MATLAB Function8/4(proj_heading_set) -> Selector9/1
  MATLAB Function8/3(proj_y_set) -> Selector8/1
  MATLAB Function8/2(proj_x_set) -> Selector7/1
  MATLAB Function8/1(match_point_index_set) -> Selector6/1
  Selector6/1 -> [origin_match_point_index]
  Selector7/1 -> [origin_x]
  Selector8/1 -> [origin_y]
  Selector9/1 -> [origin_heading]
  Selector10/1 -> [origin_kappa]
  [host_x] -> MATLAB Function8/1(x_set)
  [host_y] -> MATLAB Function8/2(y_set)
  [referenceline_y] -> MATLAB Function8/4(frenet_path_y)  "referenceline_y"
  [referenceline_x] -> MATLAB Function8/3(frenet_path_x)  "referenceline_x"
  [referenceline_heading] -> MATLAB Function8/5(frenet_path_heading)
  [referenceline_kappa] -> MATLAB Function8/6(frenet_path_kappa)
  Selector/1 -> [host_match_point_index]

== system EMPlanner_cs_old/Audi_A8_Sedan_2/Dynamics_Simple/Chassis ==
  TransmissionTorque_[Nm] : Inport
  BrakePressure_[bar] : Inport  Port=2
  DeltaSteer_[deg] : Inport  Port=3
  Initial_Vx_[m s-1] : Inport  Port=4
  Abs : Abs
  Bicycle_model_[XYZ] : Subsystem
      mask Display: image(imread('Bicycle_model.png'));
  Constant3 : Constant  Value=[0 0]
  Constant4 : Constant  Value=[0 0]
  Degrees to Radians : simulink_extras/Transformations/Degrees to Radians
  FinalDriveRatio : Gain  Gain=p.Rfd  SaturateOnIntegerOverflow=on  OutDataTypeStr=Inherit: Same as input  ParamDataTypeStr=Inherit: Same as input
  "FinalDriveRatio " : Gain  Gain=p.Rfd  SaturateOnIntegerOverflow=on  OutDataTypeStr=Inherit: Same as input  ParamDataTypeStr=Inherit: Same as input
  FrontTyre : Subsystem
      mask Display: image(imread('Tyre.png'));
  Gain : Gain  Gain=2*pi/60
  MuxDynState : Subsystem
  Power Assisted Steering : Subsystem
  Product : Product  RndMeth=Zero
  RearTyre : Subsystem
      mask Display: image(imread('Tyre.png'));
  SteerRatio : Gain  Gain=1/p.SteerRatio
  Terminator4 : Terminator
  "[ms-1 --> rpm]" : Gain  Gain=60/(2*pi*p.Rw)  SaturateOnIntegerOverflow=on  OutDataTypeStr=Inherit: Same as input  ParamDataTypeStr=Inherit: Same as input
  to_kW : Gain  Gain=0.001
  State : Outport
  VehicleSpeed_[ms-1] : Outport  Port=2
  Vy_[ms-1] : Outport  Port=3
  ax_[ms-2] : Outport  Port=4
  ay_[ms-2] : Outport  Port=5
  PDrive_[kW] : Outport  Port=6
  TransmissionOut_[rpm] : Outport  Port=7
  wires:
  [vy] -> Vy_[ms-1]/1  "vy_[ms-1]"
  to_kW/1 -> PDrive_[kW]/1  "PDrive_[kW]"
  Gain/1 -> Product/1
  Bicycle_model_[XYZ]/10(ax_[ms-2]) -> ax_[ms-2]/1  "ax_[ms-2]"
  Product/1 -> to_kW/1
  [DT] -> Product/2
  Bicycle_model_[XYZ]/11(ay_[ms-2]) -> ay_[ms-2]/1  "ay_[ms-2]"
  Abs/1 -> Bicycle_model_[XYZ]/7(|vx|_[ms-1])
  Degrees to Radians/1 -> SteerRatio/1
  [vx] -> Abs/1
  SteerRatio/1 -> [DeltaWheel], Bicycle_model_[XYZ]/1(DeltaWheel_[rad])  "DeltaWheel_[rad]"
  TransmissionTorque_[Nm]/1 -> "FinalDriveRatio "/1  "DriveTorque_[Nm]"
  RearTyre/1(FyRear_[N]) -> Bicycle_model_[XYZ]/8(Fy_rear_[N])  "Fy_rear_[N]"
  FrontTyre/1(FyFront_[N]) -> Bicycle_model_[XYZ]/9(Fy_front_[N])  "Fy_front_[N]"
  Bicycle_model_[XYZ]/1(|vx|_[ms-1]1) -> [Absvx]  "|vx|_[ms-1]"
  Bicycle_model_[XYZ]/2(vy_[ms-1]) -> [vy], MuxDynState/2(vy [ms-1])  "Vy_[ms-1]"
  Bicycle_model_[XYZ]/4(RollAngle_[rad]) -> MuxDynState/4(R [rad]), [RollAngle]  "RollAngle_[rad]"
  Bicycle_model_[XYZ]/6(YawAngle_[rads-1]) -> [YawRate]  "YawRate_[rad s-1]"
  Bicycle_model_[XYZ]/7(Vx_[ms-1]) -> [vx]  "Vx_[ms-1]"
  [DeltaWheel] -> FrontTyre/1(DeltaWheel_[rad])
  [Absvx] -> FrontTyre/2(|vx|_[ms-1])
  [vy] -> FrontTyre/3(vy_[ms-1])
  [YawRate] -> FrontTyre/4(dYawAngle_[rads-1])
  [Absvx] -> RearTyre/1(|vx|_[ms-1])
  [vy] -> RearTyre/2(vy_[ms-1])
  [YawRate] -> RearTyre/3(dpsi_[rads-1])
  Bicycle_model_[XYZ]/3(vz_[ms-1]) -> MuxDynState/3(vz [ms-1])  "Vz_[ms-1]"
  Bicycle_model_[XYZ]/8(PitchAngle_[rad]) -> MuxDynState/5(P [rad])  "PitchAngle_[rad]"
  Bicycle_model_[XYZ]/9(YawAngle_[rad]) -> MuxDynState/6(Y [rad])  "YawAngle_[rad]"
  "[ms-1 --> rpm]"/1 -> Gain/1, FinalDriveRatio/1
  FinalDriveRatio/1 -> TransmissionOut_[rpm]/1  "TransmissionOut_[rpm]"
  [vx] -> "[ms-1 --> rpm]"/1, VehicleSpeed_[ms-1]/1, MuxDynState/1(vx [ms-1])  "vx_[ms-1]"
  [vx] -> Power Assisted Steering/1(Vx_[ms-1])
  DeltaSteer_[deg]/1 -> Power Assisted Steering/2(Delta_in_[deg])
  Power Assisted Steering/1(Delta_out_[deg]) -> Degrees to Radians/1
  [RollAngle] -> FrontTyre/5(RollAngle_[rad])
  [RollAngle] -> RearTyre/4(RollAngle_[rad])
  Constant3/1 -> Bicycle_model_[XYZ]/2(zFront_[m]_dzFront_[ms-1])  "zFront_[m]_dzFront_[m s-1]"
  Constant4/1 -> Bicycle_model_[XYZ]/3(zRear_[m]_dzRear_[ms-1])  "zRear_[m]_dzRear_[m s-1]"
  BrakePressure_[bar]/1 -> Bicycle_model_[XYZ]/4(BrakePressure_[bar])  "BrakePressure_[bar]"
  "FinalDriveRatio "/1 -> Bicycle_model_[XYZ]/5(DriveTorque_[Nm]), [DT]  "DriveTorque_[Nm]"
  Initial_Vx_[m s-1]/1 -> Bicycle_model_[XYZ]/6(v0_[ms-1])  "Initial_Vx_[m s-1]"
  Bicycle_model_[XYZ]/5(RollRate_[rads-1]) -> Terminator4/1  "RollRate_[rad s-1]"
  MuxDynState/1(State) -> State/1  "State"

== system EMPlanner_cs_old/Audi_A8_Sedan_2/Dynamics_Simple/Engine ==
  ImpellerTorque_[Nm] : Inport
  Throttle_[%] : Inport  Port=2
  Configurable Subsystem : Subsystem  BlockChoice=Rate Limiter  mask{ComputationMode=ComputationMode}
      mask prompts: ComputationMode "Compuation mode:"
      mask init:
      | SetComputationMode(gcb,ComputationMode);
      settings: AttributesFormatString=%<BlockChoice>  OpenFcn=BringToFront(gcb);  MemberBlocks=Discrete Rate Limiter,Rate Limiter
      settings: TemplateBlock=|
      | PreScanSimulinkLibrary/Configurable Subsystems/TransferFunction
      | Engine/Configurable
      | Subsystem
  Configurable Subsystem1 : Subsystem  BlockChoice=Integrator  mask{ComputationMode=ComputationMode}
      mask prompts: ComputationMode "Computation mode:"
      mask init:
      | SetComputationMode(gcb,ComputationMode);
      settings: AttributesFormatString=%<BlockChoice>  OpenFcn=BringToFront(gcb);  MemberBlocks=Discrete-Time Integrator,Integrator
      settings: TemplateBlock=|
      | PreScanSimulinkLibrary/Configurable Subsystems/integral with initial condition and limts
      | for engine/Configurable
      | Subsystem
  EngineTorque : Lookup2D  RowIndex=p.thvec  ColumnIndex=p.nevec  Table=p.emap  InputSameDT=on
  Gain : Gain  Gain=2*pi/60
  Product : Product  RndMeth=Zero
  Sum : Sum  Inputs=-+  InputSameDT=on  SaturateOnIntegerOverflow=on  OutDataTypeStr=Inherit: Same as first input
  engine + impeller inertia : Gain  Gain=1/p.Iei  SaturateOnIntegerOverflow=on  OutDataTypeStr=Inherit: Same as input  ParamDataTypeStr=Inherit: Same as input
  rad|sec2rpm : Gain  Gain=60/2/pi  SaturateOnIntegerOverflow=on  OutDataTypeStr=Inherit: Same as input  ParamDataTypeStr=Inherit: Same as input
  to_kW : Gain  Gain=0.001
  nEngine_[rpm] : Outport  InitialOutput=0
  PEngine_[kW] : Outport  Port=2  InitialOutput=0
  wires:
  rad|sec2rpm/1 -> nEngine_[rpm]/1, EngineTorque/2, Gain/1  "rpm"
  engine + impeller inertia/1 -> Configurable Subsystem1/1(In1)  "rads-2"
  EngineTorque/1 -> Sum/2, Product/2
  Sum/1 -> engine + impeller inertia/1
  Configurable Subsystem1/1(Out1) -> rad|sec2rpm/1  "rads-1"
  Throttle_[%]/1 -> Configurable Subsystem/1(In1)
  ImpellerTorque_[Nm]/1 -> Sum/1
  Configurable Subsystem/1(Out1) -> EngineTorque/1
  Product/1 -> to_kW/1
  Gain/1 -> Product/1
  to_kW/1 -> PEngine_[kW]/1

== system EMPlanner_cs_old/Audi_A8_Sedan_2/Dynamics_Simple/Gear: Auto Manual ==
  note: 0; Auto = on // Manual =off
      | 1; Auto = off // Manual =on
  Auto_Manual : Inport
  Manual_Gear : Inport  Port=2
  Auto_Gear : Inport  Port=3
  If : If  IfExpression=u1 == 0
  If Action Subsystem : Subsystem  TreatAsAtomicUnit=on
  If Action Subsystem1 : Subsystem  TreatAsAtomicUnit=on
  Merge : Merge
  Gear : Outport
  wires:
  If Action Subsystem/1(Out1) -> Merge/1
  Auto_Gear/1 -> If Action Subsystem/1(In1)
  If/1 -> If Action Subsystem/Action
  Merge/1 -> Gear/1
  If Action Subsystem1/1(Out1) -> Merge/2
  Manual_Gear/1 -> If Action Subsystem1/1(In1)
  If/2 -> If Action Subsystem1/Action
  Auto_Manual/1 -> If/1

== system EMPlanner_cs_old/Audi_A8_Sedan_2/Dynamics_Simple/ShiftLogic ==
  Throttle_[%] : Inport
  GearNr_[-] : Inport  Port=2
  Auto_GearShift : Inport  Port=3
  VehSpeed_[ms-1] : Inport  Port=4
  Add2 : Sum
  Data Type Conversion1 : DataTypeConversion  OutDataTypeStr=double
  Detect Increase1 : simulink/Logic and Bit Operations/Detect Increase  vinit=0.0  OutDataTypeStr=uint8
  Detect Increase : Subsystem
  Gear limitation : Saturate  UpperLimit=p.maxGear  LowerLimit=1
  Gear limitation while shifting : Saturate  UpperLimit=p.maxGear  LowerLimit=1
  GearNeutral : Constant  Value=0
  GearReverse : Constant  Value=-1
  "IC, gear = 1" : Memory  InitialCondition=1  InheritSampleTime=on
  If Action Neutral : Subsystem  TreatAsAtomicUnit=on
  If Action Normal : Subsystem  TreatAsAtomicUnit=on
  If Action Reverse : Subsystem  TreatAsAtomicUnit=on
  Memory : Memory  InheritSampleTime=on
  Merge : Merge  Inputs=3
  Relational Operator : RelationalOperator  OutDataTypeStr=boolean  RndMeth=Nearest
  Relational Operator1 : RelationalOperator  Operator=<=  OutDataTypeStr=boolean  RndMeth=Nearest
  Shift_Down time : Delay  DelayLength=p.ShiftDown_fac
  Shift_Up time : Delay  DelayLength=p.ShiftUp_fac
  Sum : Sum  Inputs=+-
  interp_down : Lookup2D  RowIndex=p.downth  ColumnIndex=[1:p.maxGear]  Table=p.downtab  LookUpMeth=Interpolation-Use End Values  InputSameDT=on
  interp_up : Lookup2D  RowIndex=p.upth  ColumnIndex=[1:p.maxGear]  Table=p.uptab  LookUpMeth=Interpolation-Use End Values  InputSameDT=on
  reverse/neutral/normal gear : If  IfExpression=u1 == 0  ElseIfExpressions=u1 < 0
  to_ms-1 : Gain  Gain=1/3.6
  "to_ms-1 " : Gain  Gain=1/3.6
  GearNr : Outport
  wires:
  Auto_GearShift/1 -> reverse/neutral/normal gear/1
  "IC, gear = 1"/1 -> If Action Normal/1(In1)
  Merge/1 -> GearNr/1
  If Action Reverse/1(Out1) -> Merge/2
  If Action Neutral/1(Out1) -> Merge/1
  If Action Normal/1(Out1) -> Merge/3
  reverse/neutral/normal gear/3 -> If Action Normal/Action
  reverse/neutral/normal gear/1 -> If Action Neutral/Action
  reverse/neutral/normal gear/2 -> If Action Reverse/Action
  GearReverse/1 -> If Action Reverse/1(In1)
  GearNeutral/1 -> If Action Neutral/1(In1)
  Shift_Down time/1 -> Sum/2
  Shift_Up time/1 -> Sum/1
  Detect Increase/1(Out1) -> Shift_Up time/1
  Data Type Conversion1/1 -> Shift_Down time/1
  Detect Increase1/1 -> Data Type Conversion1/1
  Sum/1 -> Add2/1
  Memory/1 -> Add2/2  "GearNr_[-]"
  Add2/1 -> Gear limitation while shifting/1
  Gear limitation while shifting/1 -> "IC, gear = 1"/1, Memory/1  "GearNr_[-]"
  Throttle_[%]/1 -> interp_down/1, interp_up/1
  Relational Operator/1 -> Detect Increase/2(In2)
  Relational Operator1/1 -> Detect Increase1/1
  interp_down/1 -> "to_ms-1 "/1
  VehSpeed_[ms-1]/1 -> Relational Operator/1, Relational Operator1/1
  interp_up/1 -> to_ms-1/1
  Gear limitation/1 -> interp_down/2, interp_up/2, Detect Increase/1(GearNr_[-])
  GearNr_[-]/1 -> Gear limitation/1
  to_ms-1/1 -> Relational Operator/2
  "to_ms-1 "/1 -> Relational Operator1/2

== system EMPlanner_cs_old/Audi_A8_Sedan_2/Dynamics_Simple/Transmission ==
  nEngine_[rpm] : Inport
  GearNr_[-] : Inport  Port=2
  n_TransmissionOut_[rpm] : Inport  Port=3
  Torque_Converter : Subsystem
      mask Display: image(imread('TorqueConverter.png'));
  Transmission_Ratio : Subsystem
  Viscous coupling : Lookup  InputValues=[-5:0.1:5]*p.m/4  Table=p.m/4*tanh([-5:0.1:5])
  ImpellerTorque_[Nm] : Outport  InitialOutput=0
  TransmissionTorque_[Nm] : Outport  Port=2  InitialOutput=0
  wires:
  Torque_Converter/2(TurbineTorque_[Nm]) -> Viscous coupling/1  "Converter_Torque_[Nm]"
  Transmission_Ratio/2(nTransmissionIn_[rpm]) -> Torque_Converter/2(nTransmission_[rpm])
  nEngine_[rpm]/1 -> Torque_Converter/1(nEngine_[rpm])
  GearNr_[-]/1 -> Transmission_Ratio/2(GearNr_[-]), Torque_Converter/3(Gear nr)
  n_TransmissionOut_[rpm]/1 -> Transmission_Ratio/3(nTransmissionOut_[rpm])
  Torque_Converter/1(ImpellerTorque_[Nm]) -> ImpellerTorque_[Nm]/1
  Transmission_Ratio/1(tTransmissionOut_[Nm]) -> TransmissionTorque_[Nm]/1
  Viscous coupling/1 -> Transmission_Ratio/1(tTransmissionIn_[Nm])
